simulink model "CustomMathFunction"  (R2020a)
settings: Solver=VariableStepAuto  StartTime=0.0  StopTime=10.0  RelTol=1e-3
settings Model: Creator=Mohammad  LastModifiedBy=Mohammad

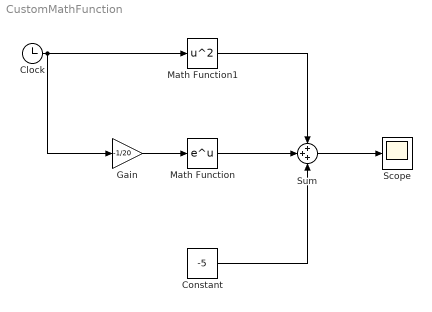
== system CustomMathFunction ==
  Clock : Clock
  Constant : Constant  Value=-5
  Gain : Gain  Gain=-1/20
  Math Function : Math  SaturateOnIntegerOverflow=on
  Math Function1 : Math  Operator=square  SaturateOnIntegerOverflow=on
  Scope : Scope
  Sum : Sum  Inputs=+++
  wires:
  Constant/1 -> Sum/3
  Math Function1/1 -> Sum/1
  Sum/1 -> Scope/1
  Math Function/1 -> Sum/2
  Clock/1 -> Gain/1, Math Function1/1
  Gain/1 -> Math Function/1
